simulink model "car_suspension_absolutedisplacements"  (R2024a)
settings: Solver=VariableStepAuto  StartTime=0.0  StopTime=5  RelTol=1e-3
values from neighbouring files (symbols this model uses):
  C1 = 700    [task1.m]
  C2 = 900    [task1.m]
  C3 = 300    [task1.m]
  K1 = 2200    [task1.m]
  K2 = 8000    [task1.m]
  K3 = 120000    [task1.m]
  M1 = 50    [task1.m]
  M2 = 250    [task1.m]
  M3 = 100    [task1.m]
settings Model: Creator=co1il  LastModifiedBy=Rotim
settings SolverCC: AlgebraicLoopSolver=TrustRegion
settings DataIOCC: ReturnWorkspaceOutputs=off
settings DebuggingCC: UnconnectedInputMsg=warning  UnconnectedOutputMsg=warning  UnconnectedLineMsg=warning  PregeneratedLibrarySubsystemCodeDiagnostic=none  ArithmeticOperatorsInVariantConditions=warning
settings ModelReferenceCC: EnableRefExpFcnMdlSchedulingChecks=on
settings SFSimCC: SimUseLocalCustomCode=off  CustomCodeUndefinedFunction=UseInterfaceOnly
settings RTWCC: RTWUseLocalCustomCode=off  GPUComputeCapability=3.5
settings CodeAppCC: StateflowObjectComments=on

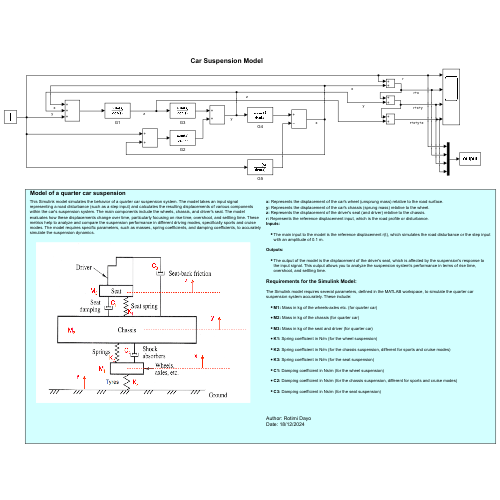
[thumbnail: Simulink's stored preview of the top-level diagram]
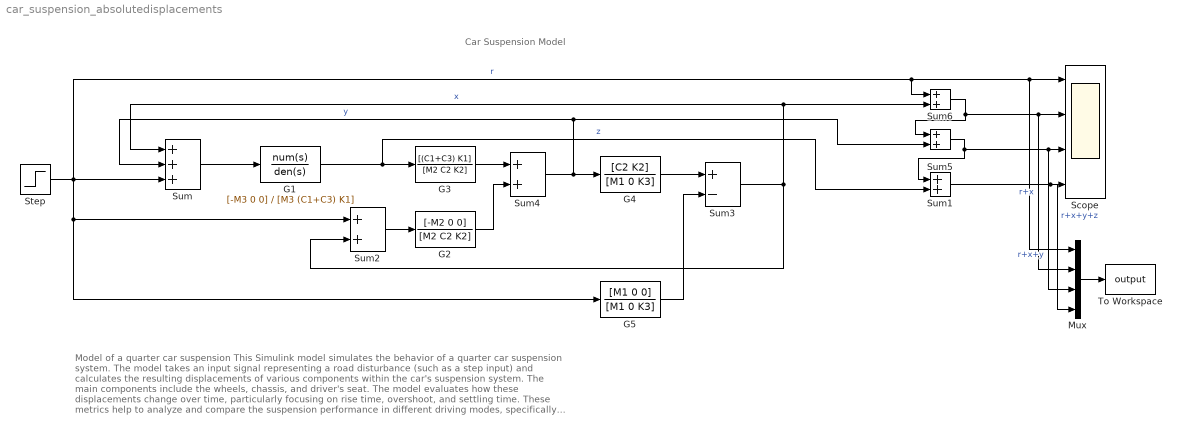
== system car_suspension_absolutedisplacements ==
  note: Model of a quarter car suspension
      |
      | This Simulink model simulates the behavior of a quarter car suspension system. The model takes an input signal representing a road disturbance (such as a step input) and calculates the resulting displacements of various components within the car's suspension system. The main components include the wheels, chassis, and driver's seat. The model evaluates how these displacements change over time, particularly focusing on rise time, overshoot, and settling time. These metrics help to analyze and compare the suspension performance in different driving modes, specifically sports and cruise modes. The model requires specific parameters, such as masses, spring coefficients, and damping coefficients, to accurately simulate the suspension dynamics.
      |
      | x: Represents the displacement of the car's wheel (unsprung mass) relative to the road surface.
      | y: Represents the displacement of the car's chassis (sprung mass) relative to the wheel.
      | z: Represents the displacement of the driver's seat (and driver) relative to the chassis.
      | r: Represents the reference displacement input, which is the road profile or disturbance.
      | Inputs:
      | The main input to the model is the reference displacement r(t), which simulates the road disturbance or the step input with an amplitude of 0.1 m.
      | Outputs:
      | The output of the model is the displacement of the driver's seat, which is affected by the suspension's response to the input signal. This output allows you to analyze the suspension system's performance in terms of rise time, overshoot, and settling time.
      | Requirements for the Simulink Model:
      | The Simulink model requires several parameters, defined in the MATLAB workspace, to simulate the quarter car suspension system accurately. These include:
      | M1: Mass in kg of the wheels-axles etc. (for quarter car)
      | M2: Mass in kg of the chassis (for quarter car)
      | M3: Mass in kg of the seat and driver (for quarter car)
      | K1: Spring coefficient in N/m (for the wheel suspension)
      | K2: Spring coefficient in N/m (for the chassis suspension, different for sports and cruise modes)
      | K3: Spring coefficient in N/m (for the seat suspension)
      | C1: Damping coefficient in Ns/m (for the wheel suspension)
      | C2: Damping coefficient in Ns/m (for the chassis suspension, different for sports and cruise modes)
      | C3: Damping coefficient in Ns/m (for the seat suspension)
      |
      | Author: Rotimi Dayo
      | Date: 18/12/2024
  note: Car Suspension Model
  G1 : TransferFcn  Numerator=[-M3 0 0]  Denominator=[M3 (C1+C3) K1]
  G2 : TransferFcn  Numerator=[-M2 0 0]  Denominator=[M2 C2 K2]
  G3 : TransferFcn  Numerator=[(C1+C3) K1]  Denominator=[M2 C2 K2]
  G4 : TransferFcn  Numerator=[C2 K2]  Denominator=[M1 0 K3]
  G5 : TransferFcn  Numerator=[M1 0 0]  Denominator=[M1 0 K3]
  Mux : Mux
  Scope : Scope  NumInputPorts=4
  Step : Step  After=0.1  SampleTime=0
  Sum : Sum  Inputs=+++
  Sum{1..2,4..6} (5 alike) : Sum
  Sum3 : Sum  Inputs=+-
  To Workspace : ToWorkspace  VariableName=output  SaveFormat=Timeseries  SampleTime=-1
  wires:
  G1/1 -> Sum1/2, G3/1  "z"
  Sum4/1 -> Sum/2, Sum5/2, G4/1  "y"
  Sum/1 -> G1/1
  Sum3/1 -> Sum6/2, Sum/1, Sum2/2  "x"
  Sum2/1 -> G2/1
  G4/1 -> Sum3/1
  G5/1 -> Sum3/2
  G2/1 -> Sum4/2
  G3/1 -> Sum4/1
  Step/1 -> Sum6/1, Mux/1, Scope/1, Sum2/1, G5/1, Sum/3  "r"
  Mux/1 -> To Workspace/1
  Sum1/1 -> Mux/4, Scope/4  "r+x+y+z"
  Sum6/1 -> Mux/2, Scope/2, Sum5/1  "r+x"
  Sum5/1 -> Sum1/1, Mux/3, Scope/3  "r+x+y"
